simulink model "Lab_5"  (R2017b)
settings: Solver=VariableStepAuto  StartTime=0.0  StopTime=simulation_time  MaxStep=0.1
values from neighbouring files (symbols this model uses):
  a = 800+R_e    (= 7178)    [main.m]
  A_i = [A_i_1, A_i_2, A_i_3]    [main.m]
  C_d = 2.2    [main.m]
  DCM_0 = eye(3)    [main.m]
  dim = [w, l, h]    [main.m]
  i = 0    [main.m]
  I_1 = M/12 * (w^2 + l^2)    (= 0.0153029225)    [main.m]
  I_2 = M/12 * (w^2 + h^2)    (= 0.0314850625)    [main.m]
  I_3 = M/12 * (l^2 + h^2)    (= 0.041787985)    [main.m]
  mu = 398600    [main.m]
  OMG = 0    [main.m]
  omg = 0    [main.m]
  phi_0 = 0.1    [main.m]
  psi_0 = 0.1    [main.m]
  q_0 = [0 1/sqrt(3) 1/sqrt(3) 1/sqrt(3)]    [main.m]
  rho = 2,82e-14    [main.m]
  theta = 0    [main.m]
  theta_0 = 0.1    [main.m]
  w1_0 = 0    [main.m]
  w2_0 = 0    [main.m]
  w3_0 = sqrt(mu/(R_e+800)^3)    [main.m]
  w_e = [0 0 0.00007291]    [main.m]
libraries: dspmathops x2, sharedutil x1, vrlib x1
settings Model: Creator=fcuzzocrea  LastModifiedBy=fcuzzocrea

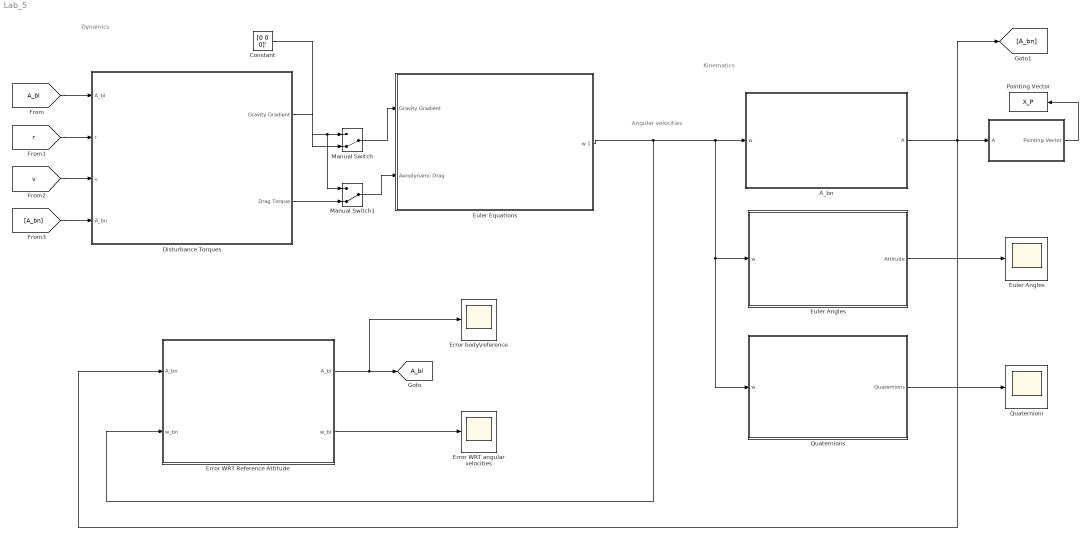
== system Lab_5 ==
  note: Dynamics
  note: Kinematics
  note: Angular velocities
  " " : Subsystem
  A_bn : Subsystem
  Constant : Constant  Value=[0 0 0]'
  Disturbance Torques : Subsystem
  "Error WRT Reference Attitude " : Subsystem
  Error WRT angular velocities : Scope
  "Error body\\reference  " : Scope
  "Euler Angles " : Subsystem
  "Euler Angles " : Scope
  "Euler Equations " : Subsystem
  Manual Switch : ManualSwitch  CurrentSetting=0
  Manual Switch1 : ManualSwitch  CurrentSetting=0
  "Pointing Vector " : ToWorkspace  VariableName=X_P  SampleTime=-1
  "Quaternioni " : Scope
  Quaternions : Subsystem
  tag scope: A_bl=global
  wires:
  A_bn/1(A) -> [A_bn], "Error WRT Reference Attitude "/1(A_bn), " "/1(A)
  " "/1("Pointing Vector ") -> "Pointing Vector "/1
  "Euler Angles "/1(Attitude) -> "Euler Angles "/1
  "Euler Equations "/1(w 1) -> "Error WRT Reference Attitude "/2(w_bn), A_bn/1(w), Quaternions/1(w), "Euler Angles "/1(w)
  "Error WRT Reference Attitude "/1(A_bl) -> "Error body\\reference  "/1, [A_bl]
  "Error WRT Reference Attitude "/2(w_bl) -> Error WRT angular velocities/1
  [A_bl] -> Disturbance Torques/1(A_bl)
  [r] -> Disturbance Torques/2(r)
  Manual Switch/1 -> "Euler Equations "/1(Gravity Gradient)
  Disturbance Torques/1("Gravity Gradient ") -> Manual Switch/2
  Constant/1 -> Manual Switch1/1, Manual Switch/1
  Quaternions/1(Quaternions) -> "Quaternioni "/1
  [v] -> Disturbance Torques/3(v)
  [A_bn] -> Disturbance Torques/4(A_bn)
  Disturbance Torques/2(Drag Torque) -> Manual Switch1/2
  Manual Switch1/1 -> "Euler Equations "/2(Aerodynamc Drag)

== system Lab_5/  ==
  A : Inport
  Constant3 : Constant  Value=[1 0 0]'  VectorParams1D=off
  Math Function : Math  Operator=transpose  SaturateOnIntegerOverflow=on
  Product1 : Product  Multiplication=Matrix(*)
  "Pointing Vector " : Outport
  wires:
  Constant3/1 -> Product1/2
  Math Function/1 -> Product1/1
  A/1 -> Math Function/1
  Product1/1 -> "Pointing Vector "/1

== system Lab_5/A_bn ==
  w : Inport
  "Assembly [w^] " : Subsystem
  Demux : Demux  Outputs=3
  Integrator : Integrator  InitialCondition=DCM_0
  MATLAB Function1 : MATLAB Function  TreatAsAtomicUnit=on
  Product : Product  Multiplication=Matrix(*)
  A : Outport
  wires:
  Product/1 -> Integrator/1
  Integrator/1 -> A/1, MATLAB Function1/1(u)
  w/1 -> Demux/1
  Demux/1 -> "Assembly [w^] "/1(w1)
  Demux/2 -> "Assembly [w^] "/2(w2)
  Demux/3 -> "Assembly [w^] "/3(w3)
  "Assembly [w^] "/1(-[w]^) -> Product/1
  MATLAB Function1/1(y) -> Product/2

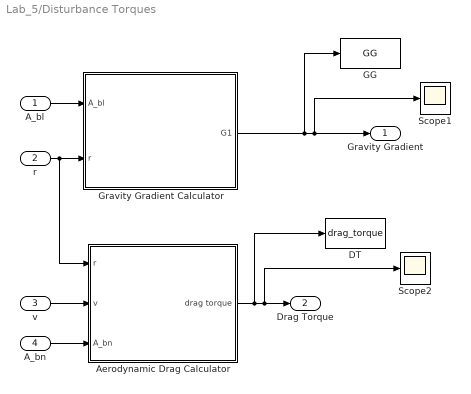
== system Lab_5/Disturbance Torques ==
  A_bl : Inport
  r : Inport  Port=2
  v : Inport  Port=3
  A_bn : Inport  Port=4
  Aerodynamic Drag Calculator : Subsystem
  DT : ToWorkspace  VariableName=drag_torque  SampleTime=-1
  GG : ToWorkspace  VariableName=GG  SampleTime=-1
  Gravity Gradient Calculator : Subsystem
  Scope1 : Scope
  Scope2 : Scope
  "Gravity Gradient " : Outport
  Drag Torque : Outport  Port=2
  wires:
  A_bl/1 -> Gravity Gradient Calculator/1(A_bl)
  r/1 -> Aerodynamic Drag Calculator/1(r), Gravity Gradient Calculator/2(r)
  Gravity Gradient Calculator/1(G1) -> GG/1, Scope1/1, "Gravity Gradient "/1
  v/1 -> Aerodynamic Drag Calculator/2(v)
  A_bn/1 -> Aerodynamic Drag Calculator/3(A_bn)
  Aerodynamic Drag Calculator/1("drag torque ") -> DT/1, Scope2/1, Drag Torque/1

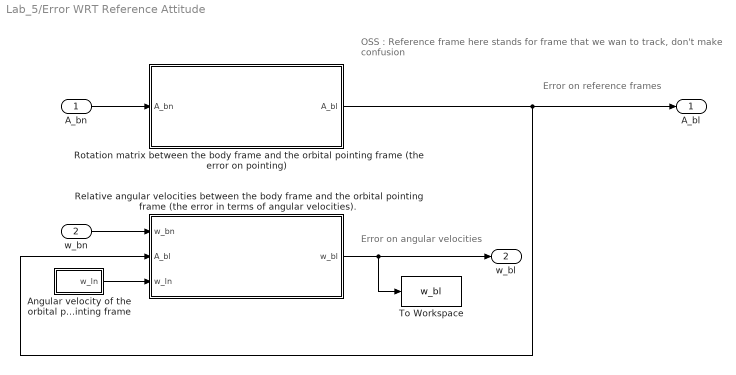
== system Lab_5/Error WRT Reference Attitude  ==
  note: Error on angular velocities
  note: Error on reference frames
  note: OSS : Reference frame here stands for frame that we wan to track, don't make confusion
  A_bn : Inport
  w_bn : Inport  Port=2
  Angular velocity of the orbital pointing frame : Subsystem
  Relative angular velocities between the body frame and the orbital pointing frame (the error in terms of angular velocities). : Subsystem
  Rotation matrix between the body frame and the orbital pointing frame (the error on pointing) : Subsystem
  To Workspace : ToWorkspace  VariableName=w_bl  SampleTime=-1
  A_bl : Outport
  w_bl : Outport  Port=2
  wires:
  A_bn/1 -> Rotation matrix between the body frame and the orbital pointing frame (the error on pointing)/1("A_bn ")
  w_bn/1 -> Relative angular velocities between the body frame and the orbital pointing frame (the error in terms of angular velocities)./1(w_bn)
  Rotation matrix between the body frame and the orbital pointing frame (the error on pointing)/1("A_bl ") -> A_bl/1, Relative angular velocities between the body frame and the orbital pointing frame (the error in terms of angular velocities)./2("A_bl ")
  Angular velocity of the orbital pointing frame/1(w_ln) -> Relative angular velocities between the body frame and the orbital pointing frame (the error in terms of angular velocities)./3("w_ln ")
  Relative angular velocities between the body frame and the orbital pointing frame (the error in terms of angular velocities)./1(w_bl) -> To Workspace/1, w_bl/1

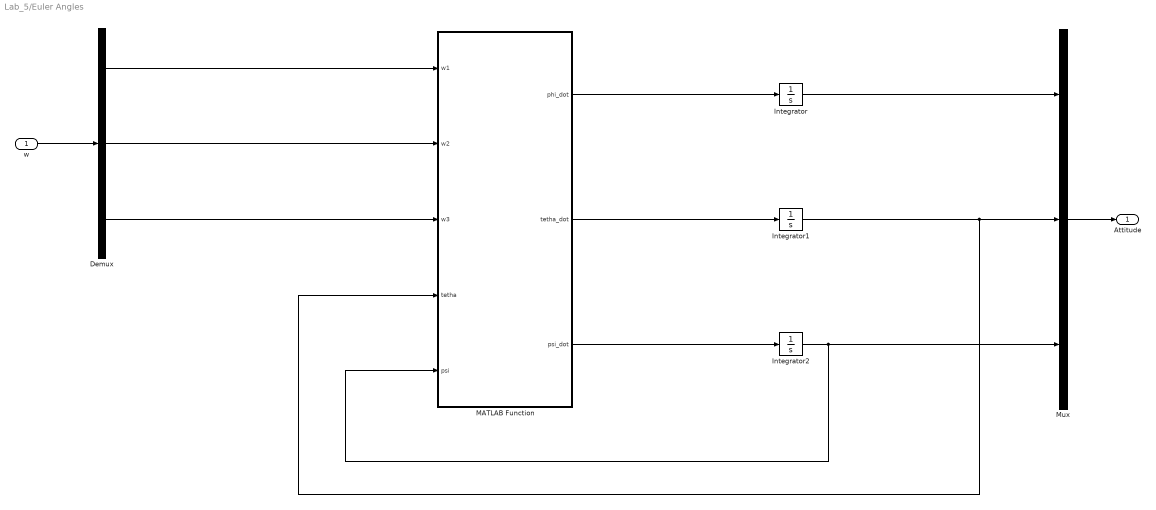
== system Lab_5/Euler Angles  ==
  w : Inport
  Demux : Demux  Outputs=3
  Integrator : Integrator  InitialCondition=phi_0
  Integrator1 : Integrator  InitialCondition=theta_0
  Integrator2 : Integrator  InitialCondition=psi_0
  MATLAB Function : MATLAB Function  TreatAsAtomicUnit=on
  Mux : Mux  Inputs=3
  Attitude : Outport
  wires:
  Demux/1 -> MATLAB Function/1(w1)
  Demux/2 -> MATLAB Function/2(w2)
  Demux/3 -> MATLAB Function/3(w3)
  MATLAB Function/1(phi_dot) -> Integrator/1
  MATLAB Function/2(tetha_dot) -> Integrator1/1
  MATLAB Function/3(psi_dot) -> Integrator2/1
  Integrator/1 -> Mux/1
  Integrator1/1 -> Mux/2, MATLAB Function/4(tetha)
  Mux/1 -> Attitude/1
  Integrator2/1 -> MATLAB Function/5(psi), Mux/3
  w/1 -> Demux/1

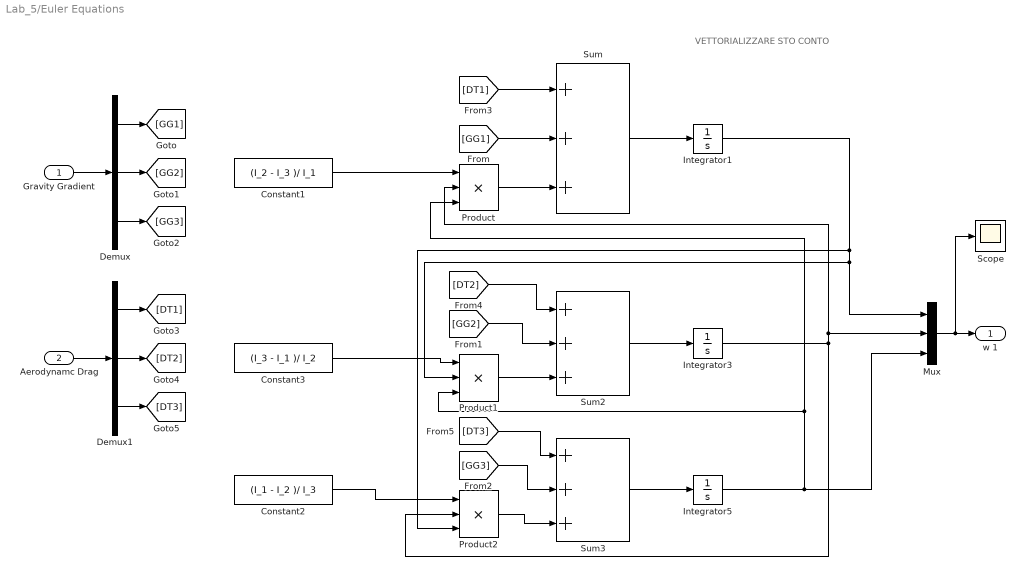
== system Lab_5/Euler Equations  ==
  note: VETTORIALIZZARE STO CONTO
  Gravity Gradient : Inport
  Aerodynamc Drag : Inport  Port=2
  Constant1 : Constant  Value=(I_2 - I_3 )/ I_1
  Constant2 : Constant  Value=(I_1 - I_2 )/ I_3
  Constant3 : Constant  Value=(I_3 - I_1 )/ I_2
  Demux : Demux  Outputs=3
  Demux1 : Demux  Outputs=3
  Integrator1 : Integrator  InitialCondition=w1_0
  Integrator3 : Integrator  InitialCondition=w2_0
  Integrator5 : Integrator  InitialCondition=w3_0
  Mux : Mux  Inputs=3
  Product : Product  Inputs=3
  Product1 : Product  Inputs=3
  Product2 : Product  Inputs=3
  Scope : Scope
  Sum : Sum  Inputs=+++
  Sum2 : Sum  Inputs=+++
  Sum3 : Sum  Inputs=+++
  w 1 : Outport
  wires:
  Integrator3/1 -> Product2/2, Mux/2, Product/2
  Integrator5/1 -> Mux/3, Product/3, Product1/3
  Constant1/1 -> Product/1
  Constant3/1 -> Product1/1
  Constant2/1 -> Product2/1
  Integrator1/1 -> Mux/1, Product1/2, Product2/3
  Mux/1 -> Scope/1, w 1/1
  [GG2] -> Sum2/2
  Sum/1 -> Integrator1/1
  Sum2/1 -> Integrator3/1
  Sum3/1 -> Integrator5/1
  Gravity Gradient/1 -> Demux/1
  Demux/1 -> [GG1]
  Demux/2 -> [GG2]
  Demux/3 -> [GG3]
  Demux1/3 -> [DT3]
  Aerodynamc Drag/1 -> Demux1/1
  Demux1/2 -> [DT2]
  Demux1/1 -> [DT1]
  Product/1 -> Sum/3
  [GG1] -> Sum/2
  [DT1] -> Sum/1
  Product1/1 -> Sum2/3
  [DT2] -> Sum2/1
  Product2/1 -> Sum3/3
  [GG3] -> Sum3/2
  [DT3] -> Sum3/1

== system Lab_5/Quaternions ==
  w : Inport
  Assmbly quaternion : Subsystem
  Demux : Demux  Outputs=3
  Gain : Gain  Gain=1/2
  Integrator : Integrator  InitialCondition=q_0
  Product : Product  Multiplication=Matrix(*)
  Quaternions : Outport
  wires:
  w/1 -> Demux/1
  Demux/1 -> Assmbly quaternion/1(w1)
  Demux/2 -> Assmbly quaternion/2(w2)
  Demux/3 -> Assmbly quaternion/3(w3)
  Assmbly quaternion/1(Q) -> Gain/1
  Gain/1 -> Product/1
  Product/1 -> Integrator/1
  Integrator/1 -> Quaternions/1, Product/2

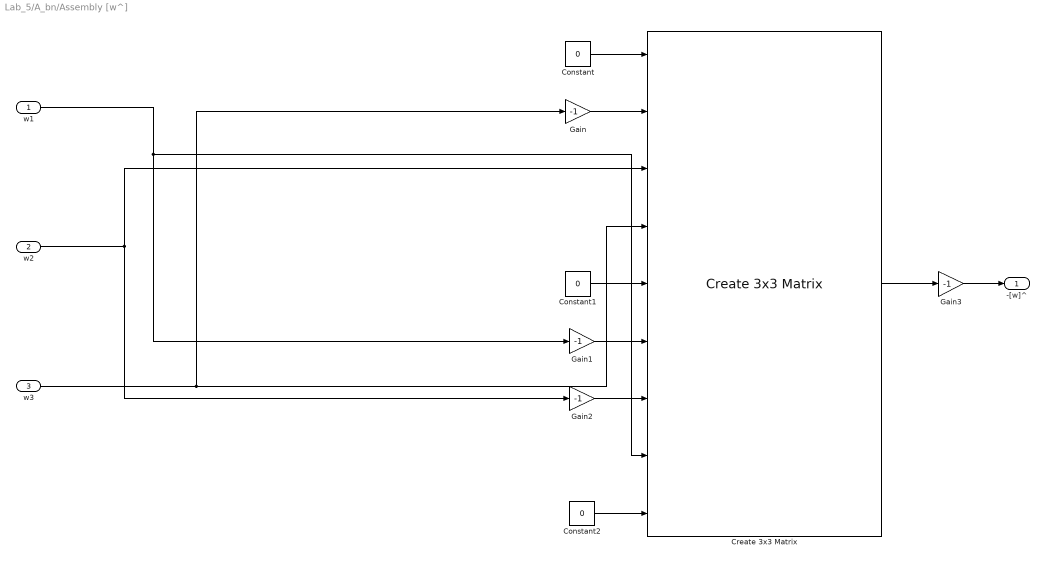
== system Lab_5/A_bn/Assembly [w^]  ==
  w1 : Inport
  w2 : Inport  Port=2
  w3 : Inport  Port=3
  Constant : Constant  Value=0
  Constant1 : Constant  Value=0
  Constant2 : Constant  Value=0
  Create 3x3 Matrix : sharedutil/Create 3x3 Matrix
  Gain{,1..3} (4 alike) : Gain  Gain=-1
  -[w]^ : Outport
  wires:
  Gain2/1 -> Create 3x3 Matrix/7
  Gain1/1 -> Create 3x3 Matrix/6
  w1/1 -> Create 3x3 Matrix/8, Gain1/1
  w3/1 -> Create 3x3 Matrix/4, Gain/1
  Constant1/1 -> Create 3x3 Matrix/5
  Constant2/1 -> Create 3x3 Matrix/9
  Constant/1 -> Create 3x3 Matrix/1
  w2/1 -> Gain2/1, Create 3x3 Matrix/3
  Gain/1 -> Create 3x3 Matrix/2
  Create 3x3 Matrix/1 -> Gain3/1
  Gain3/1 -> -[w]^/1

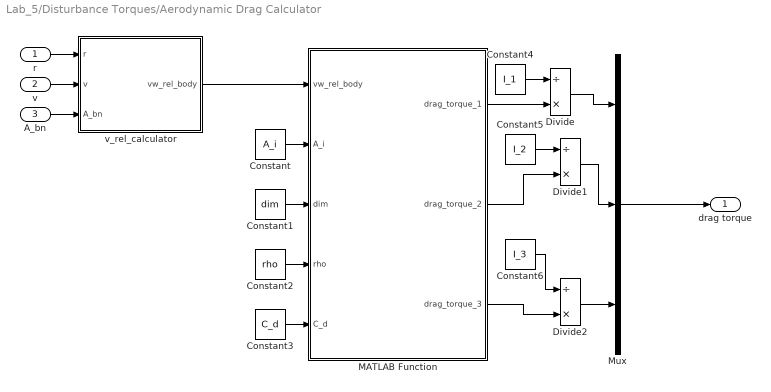
== system Lab_5/Disturbance Torques/Aerodynamic Drag Calculator ==
  r : Inport
  v : Inport  Port=2
  A_bn : Inport  Port=3
  Constant : Constant  Value=A_i
  Constant1 : Constant  Value=dim
  Constant2 : Constant  Value=rho
  Constant3 : Constant  Value=C_d
  Constant4 : Constant  Value=I_1
  Constant5 : Constant  Value=I_2
  Constant6 : Constant  Value=I_3
  Divide : Product  Inputs=/*
  Divide1 : Product  Inputs=/*
  Divide2 : Product  Inputs=/*
  MATLAB Function : MATLAB Function  TreatAsAtomicUnit=on
  Mux : Mux  Inputs=3
  v_rel_calculator : Subsystem
  "drag torque " : Outport
  wires:
  r/1 -> v_rel_calculator/1(r)
  v/1 -> v_rel_calculator/2(v)
  A_bn/1 -> v_rel_calculator/3(A_bn)
  v_rel_calculator/1(vw_rel_body) -> MATLAB Function/1(vw_rel_body)
  Constant/1 -> MATLAB Function/2(A_i)
  Constant1/1 -> MATLAB Function/3(dim)
  Constant2/1 -> MATLAB Function/4(rho)
  Constant3/1 -> MATLAB Function/5(C_d)
  Mux/1 -> "drag torque "/1
  MATLAB Function/1(drag_torque_1) -> Divide/2
  Divide/1 -> Mux/1
  Constant4/1 -> Divide/1
  Constant5/1 -> Divide1/1
  MATLAB Function/2(drag_torque_2) -> Divide1/2
  Divide1/1 -> Mux/2
  Constant6/1 -> Divide2/1
  MATLAB Function/3(drag_torque_3) -> Divide2/2
  Divide2/1 -> Mux/3

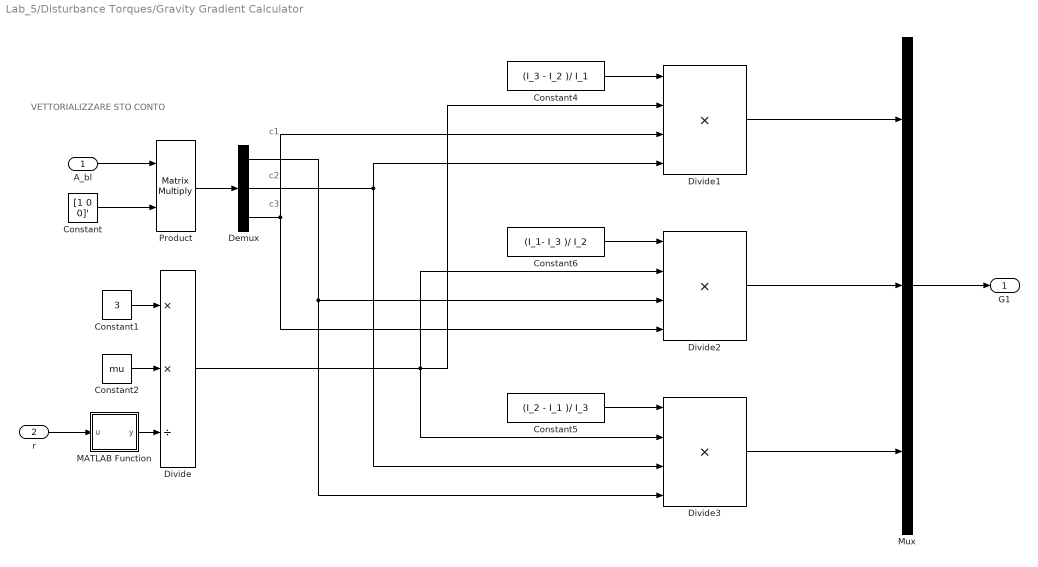
== system Lab_5/Disturbance Torques/Gravity Gradient Calculator ==
  note: VETTORIALIZZARE STO CONTO
  note: c2
  note: c3
  note: c1
  A_bl : Inport
  r : Inport  Port=2
  Constant : Constant  Value=[1 0 0]'
  Constant1 : Constant  Value=3
  Constant2 : Constant  Value=mu
  Constant4 : Constant  Value=(I_3 - I_2 )/ I_1
  Constant5 : Constant  Value=(I_2 - I_1 )/ I_3
  Constant6 : Constant  Value=(I_1- I_3 )/ I_2
  Demux : Demux  Outputs=3
  Divide : Product  Inputs=**/
  Divide1 : Product  Inputs=****
  Divide2 : Product  Inputs=****
  Divide3 : Product  Inputs=****
  MATLAB Function : MATLAB Function  TreatAsAtomicUnit=on
  Mux : Mux  Inputs=3
  Product : Product  Multiplication=Matrix(*)
  G1 : Outport
  wires:
  Demux/3 -> Divide2/4, Divide1/3
  Constant1/1 -> Divide/1
  r/1 -> MATLAB Function/1(u)
  Constant5/1 -> Divide3/1
  Divide/1 -> Divide3/2, Divide1/2, Divide2/2
  Demux/1 -> Divide3/4, Divide2/3
  Demux/2 -> Divide3/3, Divide1/4
  Product/1 -> Demux/1
  Constant6/1 -> Divide2/1
  A_bl/1 -> Product/1
  Constant4/1 -> Divide1/1
  MATLAB Function/1(y) -> Divide/3
  Constant/1 -> Product/2
  Constant2/1 -> Divide/2
  Divide1/1 -> Mux/1
  Divide2/1 -> Mux/2
  Divide3/1 -> Mux/3
  Mux/1 -> G1/1

== system Lab_5/Error WRT Reference Attitude /Angular velocity of the orbital pointing frame ==
  Derivative : Derivative
  MATLAB Function : MATLAB Function  TreatAsAtomicUnit=on
  Math Function : Math  Operator=transpose  SaturateOnIntegerOverflow=on
  Product : Product  Multiplication=Matrix(*)
  w_ln : Outport
  wires:
  [A_ln] -> Math Function/1, Derivative/1
  Math Function/1 -> Product/2
  Derivative/1 -> Product/1
  Product/1 -> MATLAB Function/1(w_ln_cross)
  MATLAB Function/1(w_ln) -> w_ln/1

== system Lab_5/Error WRT Reference Attitude /Relative angular velocities between the body frame and the orbital pointing frame (the error in terms of angular velocities). ==
  w_bn : Inport
  "A_bl " : Inport  Port=2
  "w_ln " : Inport  Port=3
  Product : Product  Multiplication=Matrix(*)
  Subtract : Sum  Inputs=+-
  w_bl : Outport
  wires:
  Product/1 -> Subtract/2
  Subtract/1 -> w_bl/1
  w_bn/1 -> Subtract/1
  "A_bl "/1 -> Product/1
  "w_ln "/1 -> Product/2

== system Lab_5/Error WRT Reference Attitude /Rotation matrix between the body frame and the orbital pointing frame (the error on pointing) ==
  note: NB : La DCM è A_bn, per cui moltiplicando A_ln * A_bn becco A_bl !!!!
  note: Reference Attitude
  "A_bn " : Inport
  Math Function1 : Math  Operator=transpose  SaturateOnIntegerOverflow=on
  Product : Product  Multiplication=Matrix(*)
  Rotation matrix between the pointing orbital frame and the inertial frame : Subsystem
  "A_bl " : Outport
  wires:
  "A_bn "/1 -> Product/1
  Rotation matrix between the pointing orbital frame and the inertial frame/1("A_L\\N ") -> Math Function1/1
  Product/1 -> "A_bl "/1
  Math Function1/1 -> Product/2

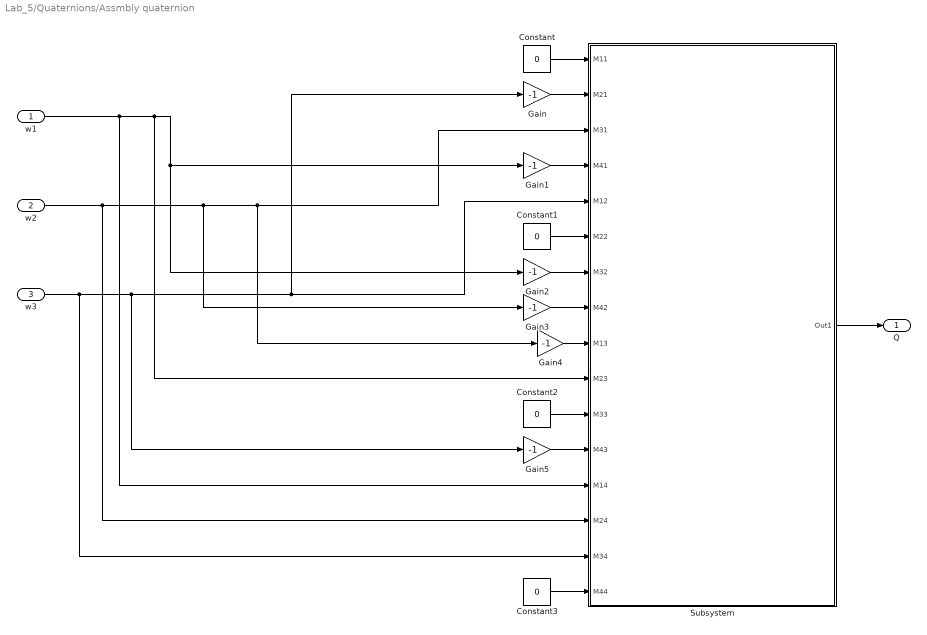
== system Lab_5/Quaternions/Assmbly quaternion ==
  w1 : Inport
  w2 : Inport  Port=2
  w3 : Inport  Port=3
  Constant{,1..3} (4 alike) : Constant  Value=0
  Gain{,1..5} (6 alike) : Gain  Gain=-1
  Subsystem : Subsystem
      mask DialogControl DescTextVar Prompt: Create 4x4 Matrix
  Q : Outport
  wires:
  Constant2/1 -> Subsystem/11(M33)
  Constant3/1 -> Subsystem/16(M44)
  Gain/1 -> Subsystem/2("M21 ")
  Gain5/1 -> Subsystem/12(M43)
  w3/1 -> Subsystem/15(M34), Gain5/1, Subsystem/5(M12), Gain/1
  Gain1/1 -> Subsystem/4("M41 ")
  Constant/1 -> Subsystem/1(M11)
  Gain2/1 -> Subsystem/7(M32)
  Constant1/1 -> Subsystem/6(M22)
  w1/1 -> Subsystem/13(M14), Subsystem/10(M23), Gain1/1, Gain2/1
  w2/1 -> Subsystem/14(M24), Gain3/1, Gain4/1, Subsystem/3("M31 ")
  Gain3/1 -> Subsystem/8(M42)
  Gain4/1 -> Subsystem/9(M13)
  Subsystem/1(Out1) -> Q/1

== system Lab_5/Disturbance Torques/Aerodynamic Drag Calculator/v_rel_calculator ==
  r : Inport
  v : Inport  Port=2
  A_bn : Inport  Port=3
  Add : Sum  Inputs=+-
  Constant : Constant  Value=w_e
  Cross Product : vrlib/Utilities/Cross Product
      settings: SourceProductBaseCode=VR
  Product : Product  Multiplication=Matrix(*)
  vw_rel_body : Outport
  wires:
  Add/1 -> Product/2
  Constant/1 -> Cross Product/1
  r/1 -> Cross Product/2
  Product/1 -> vw_rel_body/1
  v/1 -> Add/1
  A_bn/1 -> Product/1
  Cross Product/1 -> Add/2

== system Lab_5/Error WRT Reference Attitude /Rotation matrix between the body frame and the orbital pointing frame (the error on pointing)/Rotation matrix between the pointing orbital frame and the inertial frame ==
  Full Orbital Dynamics : Subsystem
  Initial Conditions (KEP) : Constant  Value=[a, e, i, OMG, omg, theta]
  Planetary Constant : Constant  Value=mu
  "A_L\\N " : Outport
  tag scope: A_ln=global
  wires:
  Planetary Constant/1 -> Full Orbital Dynamics/1(mu)
  Initial Conditions (KEP)/1 -> Full Orbital Dynamics/2(Initial Condition (kep))
  Full Orbital Dynamics/1(A_L\N) -> [A_ln], "A_L\\N "/1

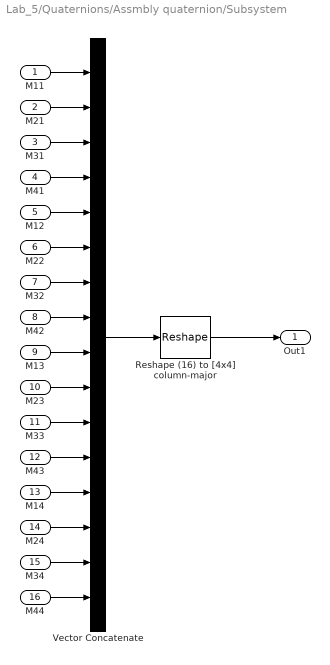
== system Lab_5/Quaternions/Assmbly quaternion/Subsystem ==
  M11 : Inport  PortDimensions=1
  "M21 " : Inport  Port=2  PortDimensions=1
  "M31 " : Inport  Port=3  PortDimensions=1
  "M41 " : Inport  Port=4  PortDimensions=1
  M12 : Inport  Port=5  PortDimensions=1
  M22 : Inport  Port=6  PortDimensions=1
  M32 : Inport  Port=7  PortDimensions=1
  M42 : Inport  Port=8  PortDimensions=1
  M13 : Inport  Port=9  PortDimensions=1
  M23 : Inport  Port=10  PortDimensions=1
  M33 : Inport  Port=11  PortDimensions=1
  M43 : Inport  Port=12  PortDimensions=1
  M14 : Inport  Port=13  PortDimensions=1
  M24 : Inport  Port=14  PortDimensions=1
  M34 : Inport  Port=15  PortDimensions=1
  M44 : Inport  Port=16  PortDimensions=1
  Reshape (16) to [4x4] column-major : Reshape  OutputDimensionality=Customize  OutputDimensions=[4,4]
  Vector Concatenate : Concatenate  NumInputs=16
  Out1 : Outport
  wires:
  M23/1 -> Vector Concatenate/10
  M44/1 -> Vector Concatenate/16
  M33/1 -> Vector Concatenate/11
  M12/1 -> Vector Concatenate/5
  M24/1 -> Vector Concatenate/14
  "M41 "/1 -> Vector Concatenate/4
  M14/1 -> Vector Concatenate/13
  M42/1 -> Vector Concatenate/8
  "M31 "/1 -> Vector Concatenate/3
  M11/1 -> Vector Concatenate/1
  M22/1 -> Vector Concatenate/6
  M34/1 -> Vector Concatenate/15
  M32/1 -> Vector Concatenate/7
  Reshape (16) to [4x4] column-major/1 -> Out1/1
  Vector Concatenate/1 -> Reshape (16) to [4x4] column-major/1
  "M21 "/1 -> Vector Concatenate/2
  M13/1 -> Vector Concatenate/9
  M43/1 -> Vector Concatenate/12

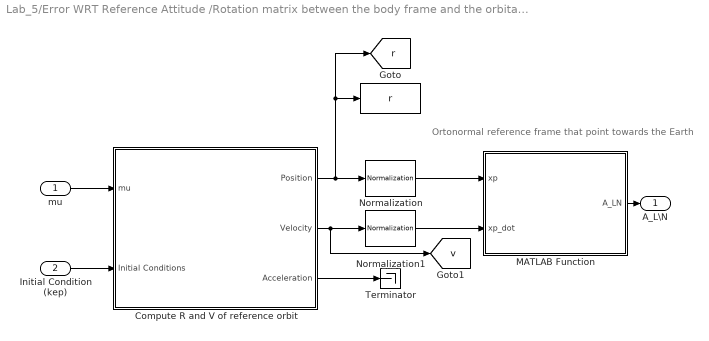
== system Lab_5/Error WRT Reference Attitude /Rotation matrix between the body frame and the orbital pointing frame (the error on pointing)/Rotation matrix between the pointing orbital frame and the inertial frame/Full Orbital Dynamics ==
  note: Ortonormal reference frame that point towards the Earth
  mu : Inport
  Initial Condition (kep) : Inport  Port=2
  " " : ToWorkspace  VariableName=r  SampleTime=-1
  Compute R and V of reference orbit : Subsystem
  MATLAB Function : MATLAB Function  TreatAsAtomicUnit=on
  Normalization : dspmathops/Normalization  NormType=2-norm  Bias=1e-10  NormOver=Each row  Dimension=1  outputDataTypeStr=Inherit: Same as product output  outputLastDataTypeStr=Inherit: Same as product output  outputMin=[]  outputMax=[]  accumDataTypeStr=Inherit: Same as product output  accumLastDataTypeStr=Inherit: Same as product output  roundingMode=Floor  overflowMode=off
      settings: SourceProductName=DSP System Toolbox
  Normalization1 : dspmathops/Normalization  NormType=2-norm  Bias=1e-10  NormOver=Each row  Dimension=1  outputDataTypeStr=Inherit: Same as product output  outputLastDataTypeStr=Inherit: Same as product output  outputMin=[]  outputMax=[]  accumDataTypeStr=Inherit: Same as product output  accumLastDataTypeStr=Inherit: Same as product output  roundingMode=Floor  overflowMode=off
      settings: SourceProductName=DSP System Toolbox
  Terminator : Terminator
  A_L\N : Outport
  tag scope: r=global, v=global
  wires:
  mu/1 -> Compute R and V of reference orbit/1(mu)
  Initial Condition (kep)/1 -> Compute R and V of reference orbit/2(Initial Conditions)
  Compute R and V of reference orbit/1(Position) -> [r], " "/1, Normalization/1
  Compute R and V of reference orbit/2(Velocity) -> [v], Normalization1/1
  Compute R and V of reference orbit/3(Acceleration) -> Terminator/1
  Normalization/1 -> MATLAB Function/1(xp)
  MATLAB Function/1(A_LN) -> A_L\N/1
  Normalization1/1 -> MATLAB Function/2(xp_dot)

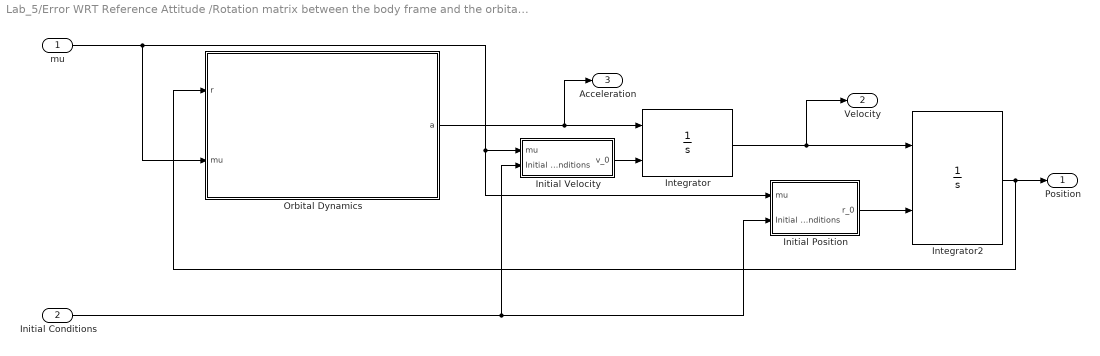
== system Lab_5/Error WRT Reference Attitude /Rotation matrix between the body frame and the orbital pointing frame (the error on pointing)/Rotation matrix between the pointing orbital frame and the inertial frame/Full Orbital Dynamics/Compute R and V of reference orbit ==
  mu : Inport
  Initial Conditions : Inport  Port=2
  Initial Position : Subsystem
  Initial Velocity : Subsystem
  Integrator : Integrator  InitialConditionSource=external  InitialCondition=[r,v]=kep2car(kep,mu);  ContinuousStateAttributes='velocity'
  Integrator2 : Integrator  InitialConditionSource=external  InitialCondition=[r,v]=kep2car(kep,mu);  ContinuousStateAttributes='position'
  Orbital Dynamics : MATLAB Function  TreatAsAtomicUnit=on
  Position : Outport
  Velocity : Outport  Port=2
  Acceleration : Outport  Port=3
  wires:
  Initial Conditions/1 -> Initial Position/2(Initial Conditions), Initial Velocity/2(Initial Conditions)
  Initial Position/1(r_0) -> Integrator2/2
  Initial Velocity/1(v_0) -> Integrator/2
  Orbital Dynamics/1(a) -> Acceleration/1, Integrator/1
  Integrator/1 -> Velocity/1, Integrator2/1
  mu/1 -> Initial Position/1(mu), Initial Velocity/1(mu), Orbital Dynamics/2(mu)
  Integrator2/1 -> Orbital Dynamics/1(r), Position/1

== system Lab_5/Error WRT Reference Attitude /Rotation matrix between the body frame and the orbital pointing frame (the error on pointing)/Rotation matrix between the pointing orbital frame and the inertial frame/Full Orbital Dynamics/Compute R and V of reference orbit/Initial Position ==
  mu : Inport
  Initial Conditions : Inport  Port=2
  MATLAB Function2 : MATLAB Function  TreatAsAtomicUnit=on
  r_0 : Outport
  wires:
  MATLAB Function2/1(r_0) -> r_0/1
  mu/1 -> MATLAB Function2/2(mu)
  Initial Conditions/1 -> MATLAB Function2/1(kep)

== system Lab_5/Error WRT Reference Attitude /Rotation matrix between the body frame and the orbital pointing frame (the error on pointing)/Rotation matrix between the pointing orbital frame and the inertial frame/Full Orbital Dynamics/Compute R and V of reference orbit/Initial Velocity ==
  mu : Inport
  Initial Conditions : Inport  Port=2
  MATLAB Function1 : MATLAB Function  TreatAsAtomicUnit=on
  v_0 : Outport
  wires:
  MATLAB Function1/1(v_0) -> v_0/1
  mu/1 -> MATLAB Function1/2(mu)
  Initial Conditions/1 -> MATLAB Function1/1(kep)

== matlab function Lab_5/Euler Angles /MATLAB Function ==
  data: phi_dot output; tetha_dot output; psi_dot output; w1 input; w2 input; w3 input; tetha input; psi input
function [phi_dot,tetha_dot, psi_dot] = euler_eqtns(w1,w2,w3, tetha, psi)

% Euler rotations (sequence 123)
phi_dot = 1/cos(tetha)*((w1*cos(psi)-w2*sin(psi)));
tetha_dot = (w2*cos(psi))+(w1*sin(psi));
psi_dot = w3 - ((w1*cos(psi) - w2*sin(psi))*(sin(tetha)/cos(tetha)));

end

== matlab function Lab_5/Error WRT Reference Attitude /Rotation matrix between the body frame and the orbital pointing frame (the error on pointing)/Rotation matrix between the pointing orbital frame and the inertial frame/Full Orbital Dynamics/Compute R and V of reference orbit/Orbital Dynamics ==
  data: r input; a output; mu input
function a  = orbit_equation(r,mu)

rn = norm(r);

a = -(mu/norm(r)^3)*r;

end

== matlab function Lab_5/A_bn/MATLAB Function1 ==
  data: u input; y output
function y = ortonormalize(u)

y = u.*3/2 - u*u'*(u./2);

y = u;

end

== matlab function Lab_5/Error WRT Reference Attitude /Rotation matrix between the body frame and the orbital pointing frame (the error on pointing)/Rotation matrix between the pointing orbital frame and the inertial frame/Full Orbital Dynamics/Compute R and V of reference orbit/Initial Velocity/MATLAB Function1 ==
  data: v_0 output; kep input; mu input
function v_0  = kep2car(kep,mu)

% Using kep2car function to find velocity at initial condition
[~,v_0]=kep2car(kep,mu);

end

== matlab function Lab_5/Error WRT Reference Attitude /Rotation matrix between the body frame and the orbital pointing frame (the error on pointing)/Rotation matrix between the pointing orbital frame and the inertial frame/Full Orbital Dynamics/Compute R and V of reference orbit/Initial Position/MATLAB Function2 ==
  data: r_0 output; kep input; mu input
function r_0  = kep2car(kep,mu)

% Using kep2car function to find position and velocity at initial condition
[r_0,~]=kep2car(kep,mu);

end

== matlab function Lab_5/Error WRT Reference Attitude /Rotation matrix between the body frame and the orbital pointing frame (the error on pointing)/Rotation matrix between the pointing orbital frame and the inertial frame/Full Orbital Dynamics/MATLAB Function ==
  data: xp input; A_LN output; xp_dot input
function A_LN = assembly_ALN(xp,xp_dot)

xp = xp';
xp_dot = xp_dot';

r_1 = xp;                                           % Points toward the Earth
r_2 = (cross(xp_dot,xp))/(norm(cross(xp_dot,xp)));  % Points toward angular momentum vector
r_3 = cross(r_1,r_2);                               % To be ortoghonal

A_LN = [r_1; r_3; r_2];                             % BE CONSISTENT WITH THE ACTUAL REFERENCE SYSTEM USED TO COMPUTE R AND V
                                                    % ACTUALLY FOR ME :
                                                    %    
                                                    %      x = direction of the vector pointing to earth    
                                                    %
                                                    %      z = direction of the out of plane vector     
                                                    %      
                                                    %      y = third vector
                                                    %

end

== matlab function Lab_5/Error WRT Reference Attitude /Angular velocity of the orbital pointing frame/MATLAB Function ==
  data: w_ln_cross input; w_ln output
function w_ln = w_component_extractor(w_ln_cross)

w_1 = w_ln_cross(3,2);
w_2 = w_ln_cross(1,3);
w_3 = w_ln_cross(2,1);

w_ln = [w_1, w_2, w_3]';
end

== matlab function Lab_5/Disturbance Torques/Gravity Gradient Calculator/MATLAB Function ==
  data: u input; y output
function y = norm3(u)

y = (norm(u))^3;

end

== matlab function Lab_5/Disturbance Torques/Aerodynamic Drag Calculator/MATLAB Function ==
  data: vw_rel_body input; drag_torque_1 output; A_i input; dim input; rho input; C_d input; drag_torque_2 output; drag_torque_3 output
function [drag_torque_1,drag_torque_2,drag_torque_3]  = aerodrag(vw_rel_body,A_i,dim,rho, C_d)

% Velocity is in km/s, we need it in m/s
vw_rel_body = vw_rel_body .* 1000;

% Define normal vectors
n_1 = [1 0 0];
n_2 = [0 1 0];
n_3 = [0 0 1];
n_4 = [-1 0 0];
n_5 = [0 -1 0];
n_6 = [0 0 -1];

% Dimensions 
w = dim(1);
l = dim(2);
h = dim(3);

% Sections 
A_i_1 = A_i(1);
A_i_2 = A_i(2);
A_i_3 = A_i(3);
A_i_4 = A_i(1);
A_i_5 = A_i(2);
A_i_6 = A_i(3);

% Distance between the center of pressure and the center of mass
r_1 = [h/2 0 0];
r_2 = [0 l/2 0];
r_3 = [0 0 w/2];
r_4 = [-h/2 0 0];
r_5 = [0 -l/2 0];
r_6 = [0 0 -w/2];

% Compute Aerodynamic Torque : reference Fundamentals of Spacecraft
% Dynamics and Control pag. 108
% Compute the dynamic pressure
dynamic_pressure = -0.5*rho*norm(vw_rel_body)*vw_rel_body;

% Compute torque due to the aerodynamic force only on face wetted by air
% If dot(n_1,vw_rel_body/norm(vw_rel_body)) <= 1 then the face is wetted
% othewise no. 
if dot(n_1,vw_rel_body/norm(vw_rel_body)) <= 1 
    F_aero_1 = dynamic_pressure * C_d * A_i_1 * dot(n_1,vw_rel_body)/norm(vw_rel_body);
    T_aero_1 = cross(r_1,F_aero_1);
else
    T_aero_1 = [0 0 0];
end

if dot(n_2,vw_rel_body/norm(vw_rel_body)) <= 1 
    F_aero_2 = dynamic_pressure * C_d * A_i_2 * dot(n_2,vw_rel_body)/norm(vw_rel_body);
    T_aero_2 = cross(r_2,F_aero_2);
else
    T_aero_2 = [0 0 0];
end

if dot(n_3,vw_rel_body/norm(vw_rel_body)) <= 1 
    F_aero_3 = dynamic_pressure * C_d * A_i_3 * dot(n_3,vw_rel_body)/norm(vw_rel_body);
    T_aero_3 = cross(r_3,F_aero_3);
else
    T_aero_3 = [0 0 0];
end

if dot(n_4,vw_rel_body/norm(vw_rel_body)) <= 1 
    F_aero_4 = dynamic_pressure * C_d * A_i_4 * dot(n_4,vw_rel_body)/norm(vw_rel_body);
    T_aero_4 = cross(r_4,F_aero_4);
else
    T_aero_4 = [0 0 0];
end

if dot(n_5,vw_rel_body/norm(vw_rel_body)) <= 1 
    F_aero_5 = dynamic_pressure * C_d * A_i_5 * dot(n_5,vw_rel_body)/norm(vw_rel_body);
    T_aero_5 = cross(r_5,F_aero_5);
else
    T_aero_5 = [0 0 0];
end

if dot(n_6,vw_rel_body/norm(vw_rel_body)) <= 1 
    F_aero_6 = dynamic_pressure * C_d * A_i_6 * dot(n_6,vw_rel_body)/norm(vw_rel_body);
    T_aero_6 = cross(r_6,F_aero_6);
else
    T_aero_6 = [0 0 0];
end

% Sum drag on all the surface
drag_torque = T_aero_1 + T_aero_2 + T_aero_3 + T_aero_4 + T_aero_5 + T_aero_5 + T_aero_6;

% We want it in components
drag_torque_1 = drag_torque(1);
drag_torque_2 = drag_torque(2);
drag_torque_3 = drag_torque(3);

end
